simulink model "model"  (Simulink 10.0)
settings: Solver=VariableStepAuto  StartTime=0.0  StopTime=48  RelTol=1e-3
values from neighbouring files (symbols this model uses):
  air_flow = 3600    [app_exported.m]    (also in skrypt.m)
  c = 1005.4    [app_exported.m]    (also in skrypt.m)
  cost = 0.27/3.6e6    (= 7.5e-08)    [app_exported.m]    (also in skrypt.m)
  lower_from = app.LowerFrom.Value    [app_exported.m]
  lower_to = app.LowerTo.Value    [app_exported.m]
  M = length * width * height * dens_air    [app_exported.m]    (also in skrypt.m = 147)
  U = U + 1/floor_res    [app_exported.m]    (also in skrypt.m = 1794240)
undefined symbols (not defined in the file or in its folder): init_temp, modulo, set_lower, set_room
libraries: simulink x2
settings Model: Creator=emilia  LastModifiedBy=Weronika
settings DataIOCC: SaveFormat=Dataset  ReturnWorkspaceOutputs=on
settings OptimizationCC: LifeSpan=auto
settings DebuggingCC: UnderspecifiedInitializationDetection=Simplified  MergeDetectMultiDrivingBlocksExec=error  SFUnexpectedBacktrackingDiag=error  SFNoUnconditionalDefaultTransitionDiag=error  SFExecutionAtInitializationDiag=warning  ArithmeticOperatorsInVariantConditions=error
settings HardwareCC: ProdBitPerPointer=64  ProdBitPerSizeT=64  ProdBitPerPtrDiffT=64  ProdLargestAtomicFloat=Float  ProdIntDivRoundTo=Zero  ProdEndianess=LittleEndian  ProdWordSize=64  ProdHWDeviceType=Intel->x86-64 (Windows64)
settings ModelReferenceCC: PropagateSignalLabelsOutOfModel=on
settings SFSimCC: SimUseLocalCustomCode=on  CustomCodeUndefinedFunction=FilterOut
settings RTWCC: RTWUseLocalCustomCode=on
settings CodeAppCC: StateflowObjectComments=off
settings GRTTargetCC: TargetLangStandard=C99 (ISO)  CombineOutputUpdateFcns=on  GRTInterface=off
settings ConfigComp: CovMetricSettings=dwe  CovHtmlReporting=off  CovSaveCumulativeToWorkspaceVar=off  CovSaveSingleToWorkspaceVar=off

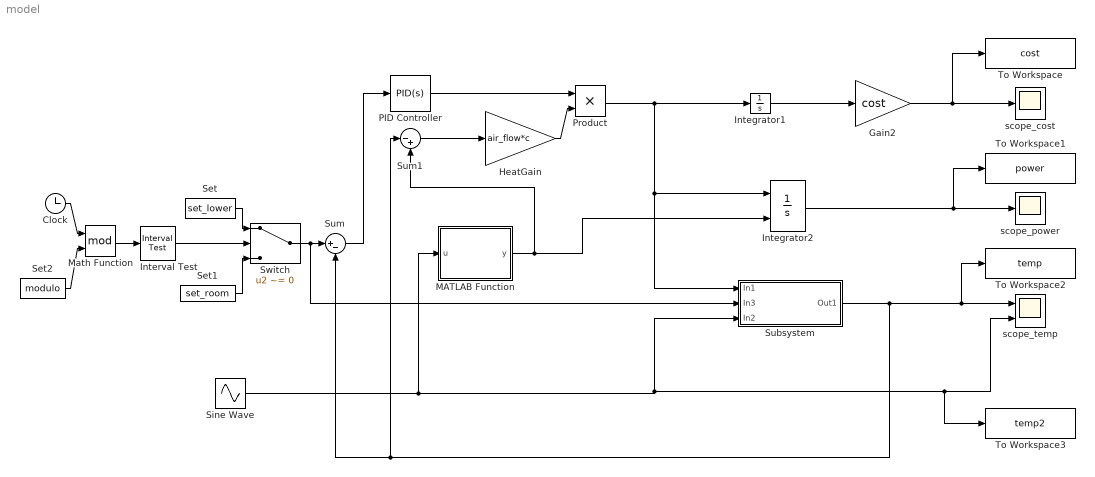
== system model ==
  Clock : Clock
  Gain2 : Gain  Gain=cost  ParamDataTypeStr=Inherit: Same as input
  HeatGain : Gain  Gain=air_flow*c
  Integrator1 : Integrator
  Integrator2 : Integrator  InitialConditionSource=external  InitialCondition=21
  Interval Test : simulink/Logic and Bit Operations/Interval Test  IntervalClosedRight=on  uplimit=lower_to  IntervalClosedLeft=on  lowlimit=lower_from  OutDataTypeStr=boolean
  MATLAB Function : MATLAB Function  TreatAsAtomicUnit=on
  Math Function : Math  Operator=mod  SignedPower=off  OutputSignalType=real  SaturateOnIntegerOverflow=on
  PID Controller : simulink/Continuous/PID Controller  Controller=PID  Form=Parallel  TimeDomain=Continuous-time  SampleTime=-1  IntegratorMethod=Forward Euler  FilterMethod=Forward Euler  ControllerParametersSource=internal  P=2  I=1.5  D=0  UseFilter=on  N=100  TunerSelectOption=Transfer Function Based (PID Tuner App)  InitialConditionSource=internal  InitialConditionForIntegrator=0  InitialConditionForFilter=0  DifferentiatorICPrevScaledInput=0  ExternalReset=none  TrackingMode=off  Kt=1  LimitOutput=off  UpperSaturationLimit=inf  LowerSaturationLimit=-inf  LinearizeAsGain=on  AntiWindupMode=none  Kb=1  POutMin=[]  POutMax=[]  IOutMin=[]  IOutMax=[]  DOutMin=[]  DOutMax=[]  NOutMin=[]  NOutMax=[]  SumOutMin=[]  SumOutMax=[]  SaturationOutMin=[]  SaturationOutMax=[]  PParamMin=[]  PParamMax=[]  IParamMin=[]  IParamMax=[]  DParamMin=[]  DParamMax=[]  NParamMin=[]  NParamMax=[]  KbParamMin=[]  KbParamMax=[]  KtParamMin=[]  KtParamMax=[]  KbOutMin=[]  KbOutMax=[]  KtOutMin=[]  KtOutMax=[]  IntegratorOutMin=[]  IntegratorOutMax=[]  FilterOutMin=[]  FilterOutMax=[]  SumI1OutMin=[]  SumI1OutMax=[]  SumI2OutMin=[]  SumI2OutMax=[]  SumI3OutMin=[]  SumI3OutMax=[]  SumI4OutMin=[]  SumI4OutMax=[]  SumDOutMin=[]  SumDOutMax=[]  DifferentiatorOutMin=[]  DifferentiatorOutMax=[]  FilterDiffOutCoefMin=[]  FilterDiffOutCoefMax=[]  ReciprocalOutMin=[]  ReciprocalOutMax=[]  SumDenOutMin=[]  SumDenOutMax=[]  SumNumOutMin=[]  SumNumOutMax=[]  DivideOutMin=[]  DivideOutMax=[]  IntegratorContinuousStateAttributes=''  IntegratorStateMustResolveToSignalObject=off  IntegratorRTWStateStorageClass=Auto  FilterContinuousStateAttributes=''  FilterStateMustResolveToSignalObject=off  FilterRTWStateStorageClass=Auto  ParallelPVariant=InternalParameters  IdealPVariant=Disabled  IVariant=InternalParameters  DVariant=InternalParameters  IntegratorVariant=Continuous  SatVariant=Disabled  AWVariant=Passthrough  PCopyVariant=Disabled  TRVariant=Disabled  FdbkBlocksVariant=Forward  IdealPFdbkVariant=Disabled  SatFdbkVariant=Disabled  DerivativeFilterVariant=ContFilter  NVariant=InternalParameters  NCopyVariant=Disabled  FilterICVariant=InternalICsFilter  IntegratorICVariant=InternalICs  ExternalResetVariant=Disabled  TRSumVariant=Passthrough  SumFdbkVariant=Disabled  SumVariant=Sum_PID
  Product : Product
  Set : Constant  Value=set_lower
  Set1 : Constant  Value=set_room
  Set2 : Constant  Value=modulo
  Sine Wave : Sin  Amplitude=6  Bias=init_temp  Frequency=2*pi/24  Phase=1.2*pi  SampleTime=0
  Subsystem : Subsystem
  Sum : Sum  Inputs=|+-
  Sum1 : Sum  Inputs=|-+
  Switch : Switch  Criteria=u2 ~= 0
  To Workspace : ToWorkspace  VariableName=cost  SaveFormat=Timeseries  SampleTime=-1
  To Workspace1 : ToWorkspace  VariableName=power  SaveFormat=Timeseries  SampleTime=-1
  To Workspace2 : ToWorkspace  VariableName=temp  SaveFormat=Timeseries  SampleTime=-1
  To Workspace3 : ToWorkspace  VariableName=temp2  SaveFormat=Timeseries  SampleTime=-1
  scope_cost : Scope
  scope_power : Scope
  scope_temp : Scope  NumInputPorts=2
  wires:
  MATLAB Function/1(y) -> Integrator2/2, Sum1/2
  Integrator2/1 -> To Workspace1/1, scope_power/1
  Product/1 -> Integrator2/1, Subsystem/1(In1), Integrator1/1
  Sum1/1 -> HeatGain/1
  Sum/1 -> PID Controller/1
  Integrator1/1 -> Gain2/1
  Sine Wave/1 -> Subsystem/3(In2), To Workspace3/1, scope_temp/2, MATLAB Function/1(u)
  PID Controller/1 -> Product/1
  Gain2/1 -> To Workspace/1, scope_cost/1
  Subsystem/1(Out1) -> To Workspace2/1, scope_temp/1, Sum1/1, Sum/2
  HeatGain/1 -> Product/2
  Clock/1 -> Math Function/1
  Math Function/1 -> Interval Test/1
  Switch/1 -> Subsystem/2(In3), Sum/1
  Set/1 -> Switch/1
  Set1/1 -> Switch/3
  Interval Test/1 -> Switch/2
  Set2/1 -> Math Function/2

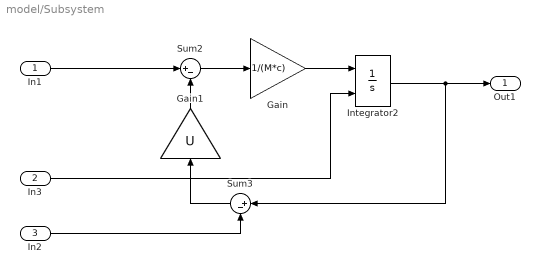
== system model/Subsystem ==
  In1 : Inport
  In3 : Inport  Port=2
  In2 : Inport  Port=3
  Gain : Gain  Gain=1/(M*c)
  Gain1 : Gain  Gain=U
  Integrator2 : Integrator  InitialConditionSource=external  InitialCondition=21
  Sum2 : Sum  Inputs=|+-
  Sum3 : Sum  Inputs=|+-
  Out1 : Outport
  wires:
  Sum3/1 -> Gain1/1
  Gain1/1 -> Sum2/2
  Integrator2/1 -> Out1/1, Sum3/1
  Gain/1 -> Integrator2/1
  In1/1 -> Sum2/1
  Sum2/1 -> Gain/1
  In2/1 -> Sum3/2
  In3/1 -> Integrator2/2

== matlab function MATLAB Function ==
  data: u input double; y output double
function y  = fcn(u)

if u<=-15
    y=75;
elseif u<=-5
    y=60;
elseif u<=0
    y=50;
elseif u<=5
    y=45;
elseif u<=15
    y=40;
else
    y=28;
end
